simulink model "PX4_Control"  (R2022b)
settings: Solver=ode1  StartTime=0.0  StopTime=inf  FixedStep=h  RelTol=1e-3  EnableMultiTasking=on
values from neighbouring files (symbols this model uses):
  h = min([h_receive,h_stream_mocap,h_send,h_optitrack,h_qualisys])    [start.m]
  h_send = 0.025    [start.m]
undefined symbols (not defined in the file or in its folder): DiscIntNeverNeededParam, Payload
libraries: Blocks x8, uavmavlinklib x2, dspnetwork x1
settings Model: SimulationMode=accelerator  Creator=dsor  LastModifiedBy=dsor
settings SolverCC: AlgebraicLoopSolver=TrustRegion  PositivePriorityOrder=on  AutoInsertRateTranBlk=on
settings OptimizationCC: BlockReduction=off  OptimizeBlockIOStorage=off  ZeroExternalMemoryAtStartup=off  ZeroInternalMemoryAtStartup=off
settings DebuggingCC: TasksWithSamePriorityMsg=none  UnconnectedInputMsg=warning  UnconnectedOutputMsg=warning  UnconnectedLineMsg=warning  SFMachineParentedDataDiag=warning
settings ModelReferenceCC: EnableRefExpFcnMdlSchedulingChecks=on
settings RTWCC: Toolchain=Simulink Real-Time Toolchain  BuildConfiguration=Faster Runs  CodeExecutionProfiling=on  TargetLang=C++  DLArmComputeVersion=19.05
settings GRTTargetCC: TargetLangStandard=C++03 (ISO)  CodeInterfacePackaging=C++ class

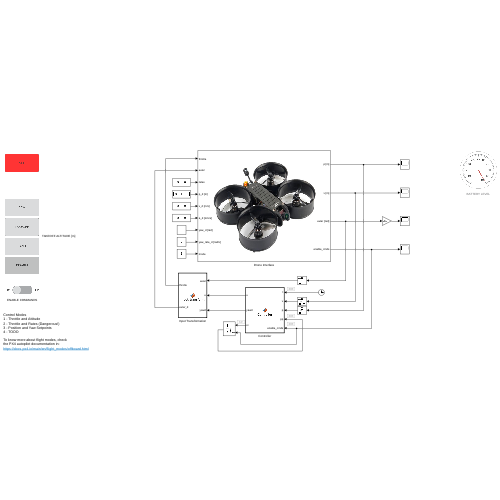
[thumbnail: Simulink's stored preview of the top-level diagram]
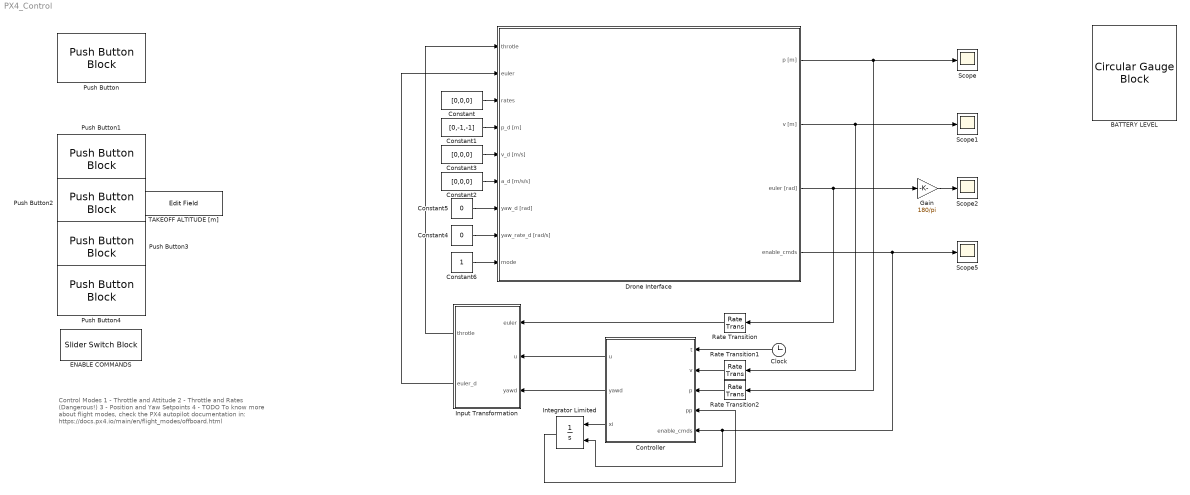
== system PX4_Control ==
  note: Control Modes
      | 1 - Throttle and Attitude
      | 2 - Throttle and Rates (Dangerous!)
      | 3 - Position and Yaw Setpoints
      | 4 - TODO
      |
      | To know more about flight modes, check
      | the PX4 autopilot documentation in:
      | https://docs.px4.io/main/en/flight_modes/offboard.html
  BATTERY LEVEL : CircularGaugeBlock  LabelPosition=Hide
  Clock : Clock
  Constant : Constant  Value=[0,0,0]
  Constant1 : Constant  Value=[0,-1,-1]
  Constant2 : Constant  Value=[0,0,0]
  Constant3 : Constant  Value=[0,0,0]
  Constant4 : Constant  Value=0
  Constant5 : Constant  Value=0
  Constant6 : Constant
  Controller : MATLAB Function  TreatAsAtomicUnit=on  SystemSampleTime=h_send
  Drone Interface : Subsystem
      mask Display: image('$imagefile'); % Use "Edit Image" on toolstrip to change.
  ENABLE COMMANDS : SliderSwitchBlock  LabelPosition=Hide
      settings: Values={{'Off', 'On'}, [0 1]}
  Gain : Gain  Gain=180/pi
  Input Transformation : MATLAB Function  TreatAsAtomicUnit=on
  Integrator Limited : Integrator  ExternalReset=either  InitialCondition=[0;0;0]  LimitOutput=on  UpperSaturationLimit=[4;4;4]  LowerSaturationLimit=-[4;4;4]
  Push Button : PushButtonBlock  ButtonText=KILL  OffValue=0.000000
  Push Button1 : PushButtonBlock  ButtonText=ARM  ButtonType=Latch  OffValue=0.000000
  Push Button2 : PushButtonBlock  ButtonText=TAKEOFF  OffValue=0.000000
  Push Button3 : PushButtonBlock  ButtonText=LAND  OffValue=0.000000
  Push Button4 : PushButtonBlock  ButtonText=DISARM  ButtonType=Latch  OffValue=0.000000
  Rate Transition : RateTransition  OutPortSampleTime=h_send
  Rate Transition1 : RateTransition  OutPortSampleTime=h_send
  Rate Transition2 : RateTransition  OutPortSampleTime=h_send
  Scope{,1..2,5} (4 alike) : Scope
  TAKEOFF ALTITUDE [m] : EditField  LabelPosition=Hide  ShowInitialText=on  Alignment=Center
  wires:
  Drone Interface/1(p [m]) -> Scope/1, Rate Transition2/1
  Drone Interface/2(v [m]) -> Scope1/1, Rate Transition1/1
  Drone Interface/3(euler [rad]) -> Rate Transition/1, Gain/1
  Constant/1 -> Drone Interface/3(rates)
  Constant1/1 -> Drone Interface/4(p_d [m])
  Constant3/1 -> Drone Interface/5(v_d [m/s])
  Constant4/1 -> Drone Interface/8(yaw_rate_d [rad/s])
  Constant5/1 -> Drone Interface/7(yaw_d [rad])
  Constant6/1 -> Drone Interface/9(mode)
  Gain/1 -> Scope2/1
  Controller/1(u) -> Input Transformation/2(u)
  Controller/2(yawd) -> Input Transformation/3(yawd)
  Constant2/1 -> Drone Interface/6(a_d [m/s/s])
  Rate Transition/1 -> Input Transformation/1(euler)
  Rate Transition1/1 -> Controller/2(v)
  Rate Transition2/1 -> Controller/3(p)
  Clock/1 -> Controller/1(t)
  Input Transformation/1(throtle) -> Drone Interface/1(throtle)
  Input Transformation/2(euler_d) -> Drone Interface/2(euler)
  Drone Interface/4(enable_cmds) -> Scope5/1, Integrator Limited/2, Controller/5(enable_cmds)
  Controller/3(xi) -> Integrator Limited/1
  Integrator Limited/1 -> Controller/4(pp)

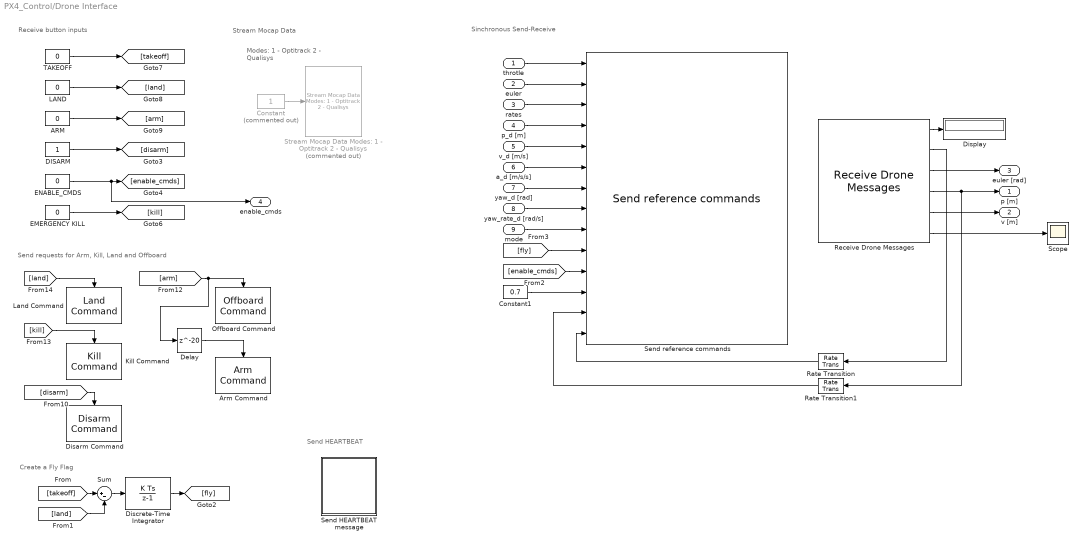
== system PX4_Control/Drone Interface ==
  note: Sinchronous Send-Receive
  note: Send HEARTBEAT
  note: Modes:
      | 1 - Optitrack
      | 2 - Qualisys
  note: Stream Mocap Data
  note: Create a Fly Flag
  note: Receive button inputs
  note: Send requests for Arm, Kill, Land and Offboard
  throtle : Inport
  euler : Inport  Port=2
  rates : Inport  Port=3
  p_d [m] : Inport  Port=4
  v_d [m/s] : Inport  Port=5
  a_d [m/s/s] : Inport  Port=6
  yaw_d [rad] : Inport  Port=7
  yaw_rate_d [rad/s] : Inport  Port=8
  mode : Inport  Port=9
  ARM : Constant  Value=0  SampleTime=h
  Arm Command : Blocks/Arm Command  SystemSampleTime=-1  VariantActivationTime=update diagram  Latency=0  AutoFrameSizeCalculation=off
  Constant : Constant  Commented=on
  Constant1 : Constant  Value=0.7
  DISARM : Constant  SampleTime=h
  Delay : Delay  DelayLength=20
  Disarm Command : Blocks/Disarm Command  SystemSampleTime=-1  VariantActivationTime=update diagram  Latency=0  AutoFrameSizeCalculation=off
  Discrete-Time Integrator : DiscreteIntegrator  gainval=1/h  SampleTime=h  LimitOutput=on  UpperSaturationLimit=1  LowerSaturationLimit=0  ICPrevOutput=DiscIntNeverNeededParam  ICPrevScaledInput=DiscIntNeverNeededParam
  Display : Display
  EMERGENCY KILL : Constant  Value=0  SampleTime=h
  ENABLE_CMDS : Constant  Value=0  SampleTime=h
  Kill Command : Blocks/Kill Command  SystemSampleTime=-1  VariantActivationTime=update diagram  Latency=0  AutoFrameSizeCalculation=off
  LAND : Constant  Value=0  SampleTime=h
  Land Command : Blocks/Land Command  SystemSampleTime=-1  VariantActivationTime=update diagram  Latency=0  AutoFrameSizeCalculation=off
  Offboard Command : Blocks/Offboard Command  SystemSampleTime=-1  VariantActivationTime=update diagram  Latency=0  AutoFrameSizeCalculation=off
  Rate Transition : RateTransition  OutPortSampleTime=h_send
  Rate Transition1 : RateTransition  OutPortSampleTime=h_send
  Receive Drone Messages : Blocks/Receive Drone Messages  SystemSampleTime=-1  VariantActivationTime=update diagram  Latency=0  AutoFrameSizeCalculation=off
  Scope : Scope
  Send HEARTBEAT message : Subsystem
  Send reference commands : Blocks/Send reference commands  SystemSampleTime=-1  VariantActivationTime=update diagram  Latency=0  AutoFrameSizeCalculation=off
  Stream Mocap Data Modes: 1 - Optitrack 2 - Qualisys : Blocks/Stream Mocap Data Modes: 1 - Optitrack 2 - Qualisys  Commented=on  SystemSampleTime=-1  VariantActivationTime=update diagram  Latency=0  AutoFrameSizeCalculation=off
  Sum : Sum  Inputs=|+-
  TAKEOFF : Constant  Value=0  SampleTime=h
  p [m] : Outport
  v [m] : Outport  Port=2
  euler [rad] : Outport  Port=3
  enable_cmds : Outport  Port=4
  wires:
  [kill] -> Kill Command/Trigger
  [land] -> Land Command/Trigger
  ENABLE_CMDS/1 -> enable_cmds/1, [enable_cmds]
  EMERGENCY KILL/1 -> [kill]
  TAKEOFF/1 -> [takeoff]
  LAND/1 -> [land]
  ARM/1 -> [arm]
  [arm] -> Delay/1, Offboard Command/Trigger
  DISARM/1 -> [disarm]
  [disarm] -> Disarm Command/Trigger
  Sum/1 -> Discrete-Time Integrator/1
  [land] -> Sum/2
  [takeoff] -> Sum/1
  Discrete-Time Integrator/1 -> [fly]
  Constant/1 -> Stream Mocap Data Modes: 1 - Optitrack 2 - Qualisys/1
  [enable_cmds] -> Send reference commands/11
  [fly] -> Send reference commands/10
  Constant1/1 -> Send reference commands/12
  mode/1 -> Send reference commands/9
  throtle/1 -> Send reference commands/1
  euler/1 -> Send reference commands/2
  rates/1 -> Send reference commands/3
  p_d [m]/1 -> Send reference commands/4
  v_d [m/s]/1 -> Send reference commands/5
  a_d [m/s/s]/1 -> Send reference commands/6
  yaw_d [rad]/1 -> Send reference commands/7
  yaw_rate_d [rad/s]/1 -> Send reference commands/8
  Rate Transition/1 -> Send reference commands/14
  Rate Transition1/1 -> Send reference commands/13
  Receive Drone Messages/1 -> Display/1
  Receive Drone Messages/3 -> euler [rad]/1
  Receive Drone Messages/4 -> Rate Transition1/1, p [m]/1
  Receive Drone Messages/5 -> v [m]/1
  Receive Drone Messages/2 -> Rate Transition/1
  Receive Drone Messages/6 -> Scope/1
  Delay/1 -> Arm Command/Trigger

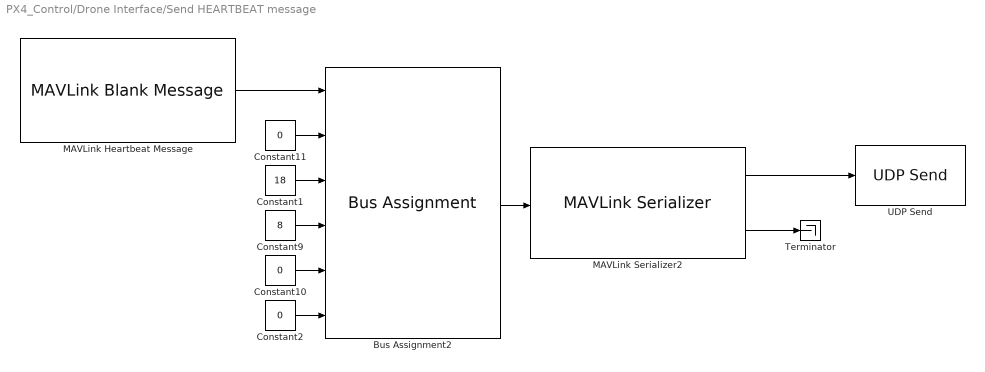
== system PX4_Control/Drone Interface/Send HEARTBEAT message ==
  Bus Assignment2 : BusAssignment  AssignedSignals=Payload.custom_mode,Payload.type,Payload.autopilot,Payload.base_mode,Payload.system_status
  Constant1 : Constant  Value=18  OutDataTypeStr=uint8  SampleTime=0.2
  Constant10 : Constant  Value=0  OutDataTypeStr=uint8  SampleTime=0.2
  Constant11 : Constant  Value=0  OutDataTypeStr=uint32  SampleTime=0.2
  Constant2 : Constant  Value=0  OutDataTypeStr=uint8  SampleTime=0.2
  Constant9 : Constant  Value=8  OutDataTypeStr=uint8  SampleTime=0.2
  MAVLink Heartbeat Message : uavmavlinklib/MAVLink Blank Message  dialectSource=Select from standard MAVLink dialects  dialect=common.xml  dialectCustom=common.xml  version=2  messageType=HEARTBEAT  SystemID=255  ComponentID=240  SampleTime=0.2
  MAVLink Serializer2 : uavmavlinklib/MAVLink Serializer  dialectSource=Select from standard MAVLink dialects  dialect=common.xml  dialectCustom=common.xml  version=2  messageType=HEARTBEAT
  Terminator : Terminator
  UDP Send : dspnetwork/UDP Send  remoteURL=Remote_IP  remotePort=Remote_Port  localURL='0.0.0.0'  localPortSource=Specify via dialog  localPort=Local_Port  sendBufferSize=8192  sampletime=-1  blockPlatform=HOST  separateLengthPort=0
      settings: LibrarySourceBlock=embeddedtargetslib/Host Communication/UDP Send
  wires:
  Bus Assignment2/1 -> MAVLink Serializer2/1
  MAVLink Heartbeat Message/1 -> Bus Assignment2/1
  MAVLink Serializer2/1 -> UDP Send/1
  MAVLink Serializer2/2 -> Terminator/1
  Constant9/1 -> Bus Assignment2/4
  Constant1/1 -> Bus Assignment2/3
  Constant11/1 -> Bus Assignment2/2
  Constant10/1 -> Bus Assignment2/5
  Constant2/1 -> Bus Assignment2/6

== matlab function PX4_Control/Controller ==
  data: t input; v input; u output; p input; pp input; yawd output; enable_cmds input; xi output
function [u,yawd,xi] = Controller(t,v,p,pp,enable_cmds)
    persistent t0;
    if isempty(t0)
        t0 = 0;
    end

    if t0 == 0 && enable_cmds == 1
        t0 = t;
    end
    if enable_cmds == 0
        t0 = 0;
    end

    tt = t-t0;
    T = 8;
    w = 2*pi/T;
    r = 1;
    yawd = 0;
    pd = [r*cos(w*tt);r*sin(w*tt);-1];
    vd = [-r*w*sin(w*tt);r*w*cos(w*tt);0];
    ad = [-r*w*w*cos(w*tt);-r*w*w*sin(w*tt);0];

    %pd = [0;-1;-0.7];
    %vd = [0;0;0];
    %ad = [0;0;0];

    Kv = 4;
    Kp = 4;
    Ki = 0.3;
    u = -Kv*(v-vd) - Kp*(p-pd) - Ki*pp + ad;
    u = u(:);

    if enable_cmds == 1
        xi = p-pd;
    else
        xi = [0;0;0];
    end

== matlab function PX4_Control/Input Transformation ==
  data: euler input; u input; throtle output; yawd input; euler_d output
function [throtle,euler_d] = input_transform(euler,u,yawd)

    persistent m g a b c d th
    if isempty(m)
        g = 9.80665;

        %%% For the IRIS drone (simulation)
        m = 1.52;
        a = 34.068;    
        b = 7.1202;
        c = 0.0074158;
        th = @(thrust) 1.7/1.52*(-b+sqrt(b*b-4*a*(c-thrust)))/(2*a);
    
        %&& For the IntelAero drone
        %m = 1.38;  % IntelAero
        %a = 8.84;
        %b = 2.955;
        %c = -1.478;
        %d = 10.37;
        %throtle =@(thrust) (tan((thrust-d)/a)-c)/b;
    
        %%% For the SnapDragon6 drone
        %m = 0.56;  % SnapDragon
        %a = 0.1377;
        %b = 0.003759;
        %c = -0.02976;
        %d = -0.05973;
        %throtle = @(thrust) 0.245/0.345*(a*exp(-c*thrust)*sqrt(thrust) + b*thrust + d);
    
        %%% For the CineWhoop drone
        %m = 0.39;
        %a = 0.0001531; 
        %b = -0.002836;
        %c = 0.07347;
        %d = -0.003982;
        %throtle = @(thrust) a*thrust*thrust*thrust + b*thrust*thrust+ c*thrust + d;
    end
    
    % Saturate the accelaration
    u(u>4) = 8;
    u(u<-4) = -8;

    % Compute pitch, roll and throtle
    Rz = eul2rotm([euler(3),0,0],'ZYX');
    T = m*Rz'*(g*[0;0;1]-u);
    pitchd = atan2(T(1),T(3));
    rolld = atan2(-T(2),norm(T([1,3])));
    throtle = th(norm(T));
    if throtle > 1
        throtle = 1;
    elseif throtle < 0
        throtle = 0;
    end

    euler_d = [yawd;pitchd;rolld];
